simulink model "AuM_HA_05_A2"  (R2020a)
settings: Solver=VariableStepAuto  StartTime=0.0  StopTime=0.2  FixedStep=1e-8  MaxStep=1e-4  MinStep=1e-9  RelTol=1e-10  EnableMultiTasking=on
values from neighbouring files (symbols this model uses):
  f_PWM = 16000    [AuM_HA05_A1_init.m]    (also in AuM_HA05_A2_init.m)
  J = 450e-6    (= 0.00045)    [AuM_HA05_A1_init.m]    (also in AuM_HA05_A2_init.m)
  K_pi = (T_oi.^2+T_S.^2)/(2/R_S*T_oi*T_S)    [AuM_HA05_A1_init.m]    (also in AuM_HA05_A2_init.m)
  L_S = 4e-3    (= 0.004)    [AuM_HA05_A1_init.m]    (also in AuM_HA05_A2_init.m)
  p = 5    [AuM_HA05_A1_init.m]    (also in AuM_HA05_A2_init.m)
  Psi_P = 4.5e-3    (= 0.0045)    [AuM_HA05_A1_init.m]    (also in AuM_HA05_A2_init.m)
  R_S = 0.58    [AuM_HA05_A1_init.m]    (also in AuM_HA05_A2_init.m)
  T_mi = 50e-6    (= 5e-05)    [AuM_HA05_A1_init.m]    (also in AuM_HA05_A2_init.m)
  T_mw = 908e-6    (= 0.000908)    [AuM_HA05_A1_init.m]    (also in AuM_HA05_A2_init.m)
  T_ni = 4*T_oi*T_S*(T_oi.^2+T_S.^2)/(T_oi+T_S).^3    [AuM_HA05_A1_init.m]    (also in AuM_HA05_A2_init.m)
  T_S = L_S/R_S    (= 0.00689655172414)    [AuM_HA05_A1_init.m]    (also in AuM_HA05_A2_init.m)
  T_SR = 50e-6    (= 5e-05)    [AuM_HA05_A1_init.m]    (also in AuM_HA05_A2_init.m)
  U_d = 24    [AuM_HA05_A1_init.m]    (also in AuM_HA05_A2_init.m)
undefined symbols (not defined in the file or in its folder): magnitude
libraries: simulink x1
settings Model: Creator=junglas  LastModifiedBy=Ravi Plenzdorf
settings SolverCC: MaxConsecutiveZCs=10000  ZeroCrossAlgorithm=Adaptive
settings DataIOCC: ReturnWorkspaceOutputs=off
settings OptimizationCC: LifeSpan=inf
settings DebuggingCC: SFUnexpectedBacktrackingDiag=warning  SFNoUnconditionalDefaultTransitionDiag=warning  SFExecutionAtInitializationDiag=none  ArithmeticOperatorsInVariantConditions=warning
settings SFSimCC: SimUseLocalCustomCode=off  CustomCodeUndefinedFunction=UseInterfaceOnly
settings RTWCC: RTWUseLocalCustomCode=off
settings CodeAppCC: StateflowObjectComments=on
settings GRTTargetCC: TargetLangStandard=C89/C90 (ANSI)
settings ConfigComp: CovMetricSettings=dw  CovHtmlReporting=on  CovSaveCumulativeToWorkspaceVar=on  CovSaveSingleToWorkspaceVar=on  CovExternalEMLEnable=off

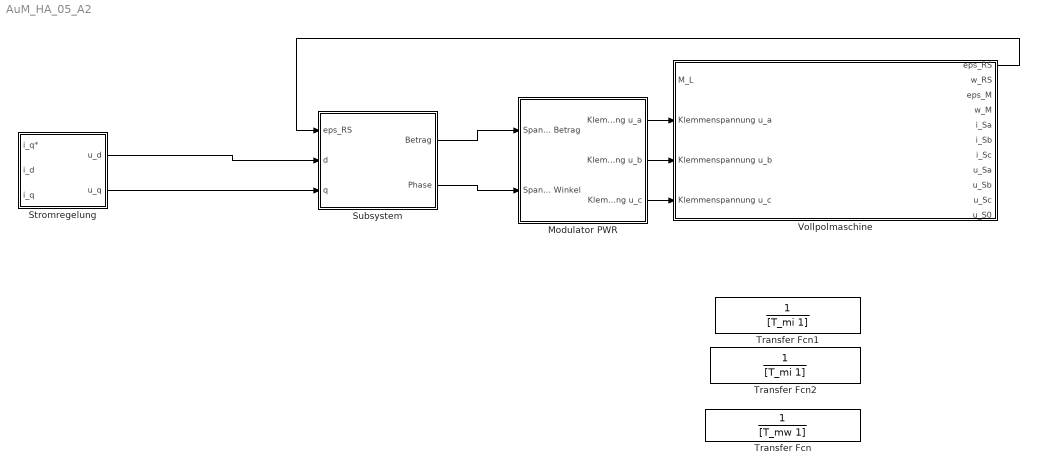
== system AuM_HA_05_A2 ==
  Modulator PWR : Subsystem  SystemSampleTime=1/1e6
  Stromregelung : Subsystem
  Subsystem : Subsystem
  Transfer Fcn : TransferFcn  Denominator=[T_mw 1]
  Transfer Fcn1 : TransferFcn  Denominator=[T_mi 1]
  Transfer Fcn2 : TransferFcn  Denominator=[T_mi 1]
  Vollpolmaschine : Subsystem
      mask Display: image('Motor_Symbol.png'); % Use "Edit Image" on toolstrip to change.
  wires:
  Modulator PWR/1(Klemmenspannung u_a) -> Vollpolmaschine/2(Klemmenspannung u_a)
  Modulator PWR/2(Klemmenspannung u_b) -> Vollpolmaschine/3(Klemmenspannung u_b)
  Modulator PWR/3(Klemmenspannung u_c) -> Vollpolmaschine/4(Klemmenspannung u_c)
  Vollpolmaschine/1(eps_RS) -> Subsystem/1(eps_RS)
  Stromregelung/1(u_d) -> Subsystem/2(d)
  Stromregelung/2(u_q) -> Subsystem/3(q)
  Subsystem/2(Phase) -> Modulator PWR/2(Spannung Winkel)
  Subsystem/1(Betrag) -> Modulator PWR/1(Spannung Betrag)

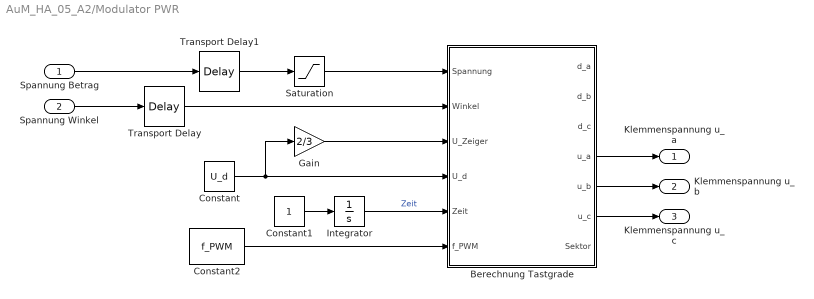
== system AuM_HA_05_A2/Modulator PWR ==
  Spannung Betrag : Inport
  Spannung Winkel : Inport  Port=2
  Berechnung Tastgrade : MATLAB Function  SystemSampleTime=1e-6
  Constant : Constant  Value=U_d
  Constant1 : Constant
  Constant2 : Constant  Value=f_PWM
  Gain : Gain  Gain=2/3
  Integrator : Integrator
  Saturation : Saturate  UpperLimit=U_d*sqrt(3)/2  LowerLimit=0
  Transport Delay : TransportDelay  DelayTime=T_SR
  Transport Delay1 : TransportDelay  DelayTime=T_SR
  Klemmenspannung u_a : Outport  VectorParamsAs1DForOutWhenUnconnected=off
  Klemmenspannung u_b : Outport  Port=2  VectorParamsAs1DForOutWhenUnconnected=off
  Klemmenspannung u_c : Outport  Port=3  VectorParamsAs1DForOutWhenUnconnected=off
  wires:
  Spannung Betrag/1 -> Transport Delay1/1
  Integrator/1 -> Berechnung Tastgrade/5(Zeit)  "Zeit"
  Constant/1 -> Berechnung Tastgrade/4(U_d), Gain/1
  Gain/1 -> Berechnung Tastgrade/3(U_Zeiger)
  Berechnung Tastgrade/6(u_c) -> Klemmenspannung u_c/1
  Berechnung Tastgrade/5(u_b) -> Klemmenspannung u_b/1
  Berechnung Tastgrade/4(u_a) -> Klemmenspannung u_a/1
  Saturation/1 -> Berechnung Tastgrade/1(Spannung)
  Constant1/1 -> Integrator/1
  Constant2/1 -> Berechnung Tastgrade/6(f_PWM)
  Spannung Winkel/1 -> Transport Delay/1
  Transport Delay/1 -> Berechnung Tastgrade/2(Winkel)
  Transport Delay1/1 -> Saturation/1

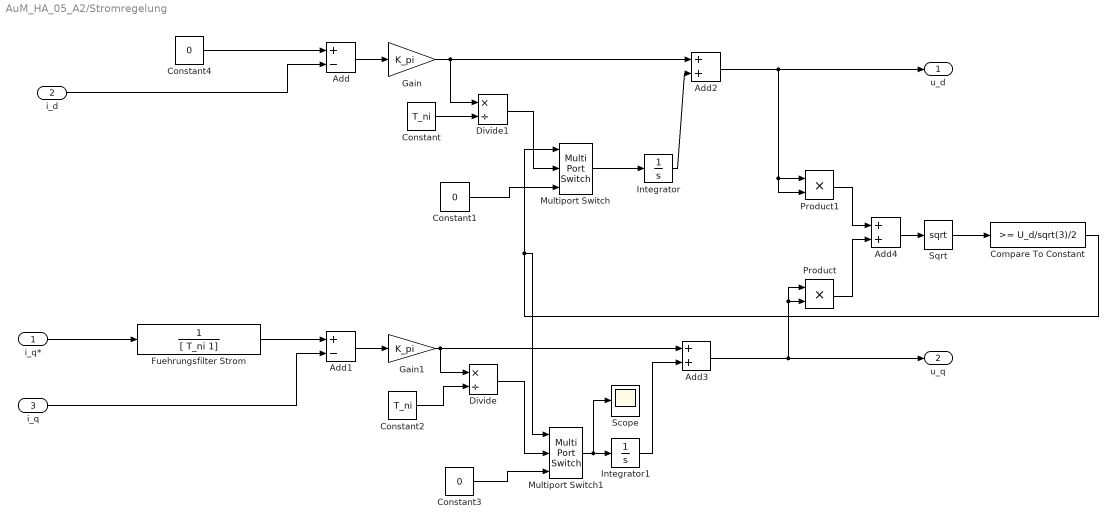
== system AuM_HA_05_A2/Stromregelung ==
  i_q* : Inport
  i_d : Inport  Port=2
  i_q : Inport  Port=3
  Add : Sum  Inputs=+-
  Add1 : Sum  Inputs=+-
  Add2 : Sum
  Add3 : Sum
  Add4 : Sum
  Compare To Constant : simulink/Logic and Bit Operations/Compare To Constant  relop=>=  const=U_d/sqrt(3)/2  OutDataTypeStr=boolean
  Constant : Constant  Value=T_ni
  Constant1 : Constant  Value=0
  Constant2 : Constant  Value=T_ni
  Constant3 : Constant  Value=0
  Constant4 : Constant  Value=0
  Divide : Product  Inputs=*/
  Divide1 : Product  Inputs=*/
  Fuehrungsfilter Strom : TransferFcn  Denominator=[ T_ni 1]
  Gain : Gain  Gain=K_pi
  Gain1 : Gain  Gain=K_pi
  Integrator : Integrator
  Integrator1 : Integrator
  Multiport Switch : MultiPortSwitch  DataPortOrder=Specify indices  DataPortIndices={0,1}
  Multiport Switch1 : MultiPortSwitch  DataPortOrder=Specify indices  DataPortIndices={0,1}
  Product : Product
  Product1 : Product
  Scope : Scope
  Sqrt : Sqrt  SaturateOnIntegerOverflow=on
  u_d : Outport  VectorParamsAs1DForOutWhenUnconnected=off
  u_q : Outport  Port=2  VectorParamsAs1DForOutWhenUnconnected=off
  wires:
  i_q/1 -> Add1/2
  i_d/1 -> Add/2
  Add1/1 -> Gain1/1
  Add/1 -> Gain/1
  i_q*/1 -> Fuehrungsfilter Strom/1
  Gain/1 -> Add2/1, Divide1/1
  Integrator/1 -> Add2/2
  Integrator1/1 -> Add3/2
  Gain1/1 -> Divide/1, Add3/1
  Constant/1 -> Divide1/2
  Multiport Switch/1 -> Integrator/1
  Constant2/1 -> Divide/2
  Multiport Switch1/1 -> Scope/1, Integrator1/1
  Add2/1 -> Product1/2, Product1/1, u_d/1
  Add3/1 -> Product/1, Product/2, u_q/1
  Constant4/1 -> Add/1
  Constant3/1 -> Multiport Switch1/3
  Divide/1 -> Multiport Switch1/2
  Divide1/1 -> Multiport Switch/2
  Constant1/1 -> Multiport Switch/3
  Compare To Constant/1 -> Multiport Switch1/1, Multiport Switch/1
  Fuehrungsfilter Strom/1 -> Add1/1
  Product/1 -> Add4/2
  Product1/1 -> Add4/1
  Add4/1 -> Sqrt/1
  Sqrt/1 -> Compare To Constant/1

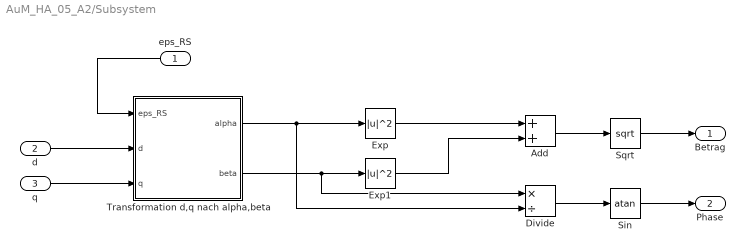
== system AuM_HA_05_A2/Subsystem ==
  eps_RS : Inport
  d : Inport  Port=2
  q : Inport  Port=3
  Add : Sum
  Divide : Product  Inputs=*/
  Exp : Math  Operator=magnitude^2  SaturateOnIntegerOverflow=on
  Exp1 : Math  Operator=magnitude^2  SaturateOnIntegerOverflow=on
  Sin : Trigonometry  Operator=atan
  Sqrt : Sqrt  SaturateOnIntegerOverflow=on
  Transformation d,q nach alpha,beta : MATLAB Function  TreatAsAtomicUnit=on
  Betrag : Outport
  Phase : Outport  Port=2
  wires:
  Exp1/1 -> Add/2
  Transformation d,q nach alpha,beta/2(beta) -> Exp1/1, Divide/1
  Transformation d,q nach alpha,beta/1(alpha) -> Divide/2, Exp/1
  Exp/1 -> Add/1
  Add/1 -> Sqrt/1
  eps_RS/1 -> Transformation d,q nach alpha,beta/1(eps_RS)
  q/1 -> Transformation d,q nach alpha,beta/3(q)
  d/1 -> Transformation d,q nach alpha,beta/2(d)
  Sqrt/1 -> Betrag/1
  Divide/1 -> Sin/1
  Sin/1 -> Phase/1

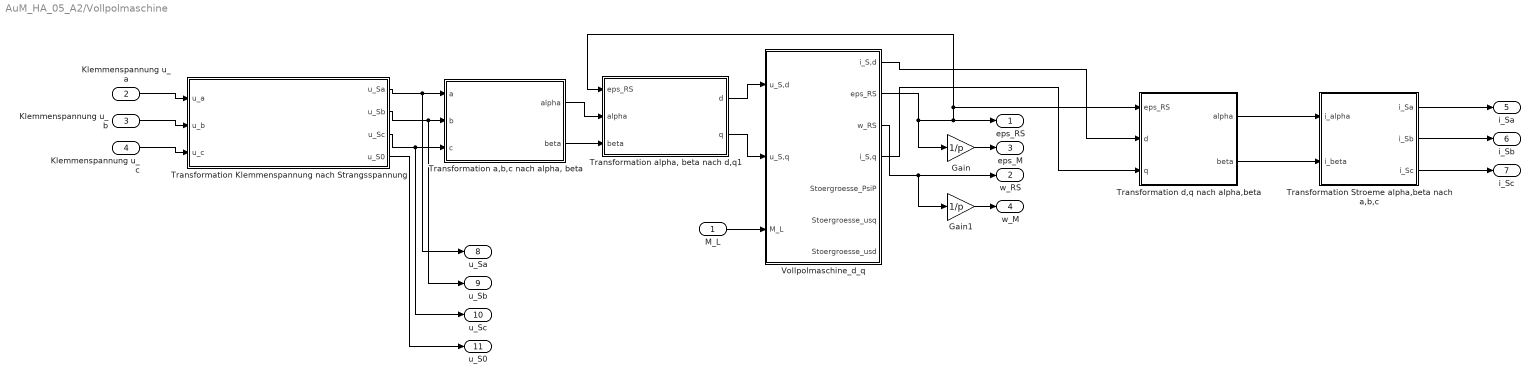
== system AuM_HA_05_A2/Vollpolmaschine ==
  M_L : Inport
  Klemmenspannung u_a : Inport  Port=2
  Klemmenspannung u_b : Inport  Port=3
  Klemmenspannung u_c : Inport  Port=4
  Gain : Gain  Gain=1/p
  Gain1 : Gain  Gain=1/p
  Transformation Klemmenspannung nach Strangsspannung : MATLAB Function  TreatAsAtomicUnit=on
  Transformation Stroeme alpha,beta nach a,b,c : MATLAB Function  TreatAsAtomicUnit=on
  "Transformation a,b,c nach alpha, beta" : MATLAB Function  TreatAsAtomicUnit=on
  "Transformation alpha, beta nach d,q1" : MATLAB Function  TreatAsAtomicUnit=on
  Transformation d,q nach alpha,beta : MATLAB Function  TreatAsAtomicUnit=on
  Vollpolmaschine_d_q : Subsystem
  eps_RS : Outport  VectorParamsAs1DForOutWhenUnconnected=off
  w_RS : Outport  Port=2  VectorParamsAs1DForOutWhenUnconnected=off
  eps_M : Outport  Port=3  VectorParamsAs1DForOutWhenUnconnected=off
  w_M : Outport  Port=4  VectorParamsAs1DForOutWhenUnconnected=off
  i_Sa : Outport  Port=5  VectorParamsAs1DForOutWhenUnconnected=off
  i_Sb : Outport  Port=6  VectorParamsAs1DForOutWhenUnconnected=off
  i_Sc : Outport  Port=7  VectorParamsAs1DForOutWhenUnconnected=off
  u_Sa : Outport  Port=8  VectorParamsAs1DForOutWhenUnconnected=off
  u_Sb : Outport  Port=9  VectorParamsAs1DForOutWhenUnconnected=off
  u_Sc : Outport  Port=10  VectorParamsAs1DForOutWhenUnconnected=off
  u_S0 : Outport  Port=11  VectorParamsAs1DForOutWhenUnconnected=off
  wires:
  Vollpolmaschine_d_q/4(i_S,q) -> Transformation d,q nach alpha,beta/3(q)
  Vollpolmaschine_d_q/1(i_S,d) -> Transformation d,q nach alpha,beta/2(d)
  Transformation Klemmenspannung nach Strangsspannung/2(u_Sb) -> u_Sb/1, "Transformation a,b,c nach alpha, beta"/2(b)
  Vollpolmaschine_d_q/3(w_RS) -> Gain1/1, w_RS/1
  Transformation Klemmenspannung nach Strangsspannung/1(u_Sa) -> u_Sa/1, "Transformation a,b,c nach alpha, beta"/1(a)
  Vollpolmaschine_d_q/2(eps_RS) -> eps_RS/1, Transformation d,q nach alpha,beta/1(eps_RS), "Transformation alpha, beta nach d,q1"/1(eps_RS), Gain/1
  Transformation Klemmenspannung nach Strangsspannung/3(u_Sc) -> "Transformation a,b,c nach alpha, beta"/3(c), u_Sc/1
  M_L/1 -> Vollpolmaschine_d_q/3(M_L)
  "Transformation a,b,c nach alpha, beta"/1(alpha) -> "Transformation alpha, beta nach d,q1"/2(alpha)
  "Transformation a,b,c nach alpha, beta"/2(beta) -> "Transformation alpha, beta nach d,q1"/3(beta)
  "Transformation alpha, beta nach d,q1"/2(q) -> Vollpolmaschine_d_q/2(u_S,q)
  Klemmenspannung u_a/1 -> Transformation Klemmenspannung nach Strangsspannung/1(u_a)
  Klemmenspannung u_b/1 -> Transformation Klemmenspannung nach Strangsspannung/2(u_b)
  Klemmenspannung u_c/1 -> Transformation Klemmenspannung nach Strangsspannung/3(u_c)
  Gain/1 -> eps_M/1
  Gain1/1 -> w_M/1
  "Transformation alpha, beta nach d,q1"/1(d) -> Vollpolmaschine_d_q/1(u_S,d)
  Transformation d,q nach alpha,beta/1(alpha) -> Transformation Stroeme alpha,beta nach a,b,c/1(i_alpha)
  Transformation d,q nach alpha,beta/2(beta) -> Transformation Stroeme alpha,beta nach a,b,c/2(i_beta)
  Transformation Stroeme alpha,beta nach a,b,c/1(i_Sa) -> i_Sa/1
  Transformation Stroeme alpha,beta nach a,b,c/2(i_Sb) -> i_Sb/1
  Transformation Stroeme alpha,beta nach a,b,c/3(i_Sc) -> i_Sc/1
  Transformation Klemmenspannung nach Strangsspannung/4(u_S0) -> u_S0/1

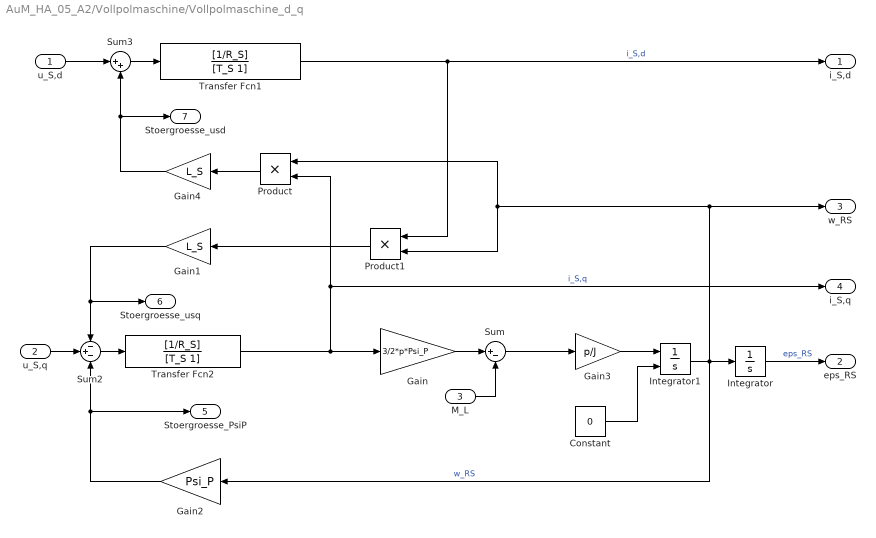
== system AuM_HA_05_A2/Vollpolmaschine/Vollpolmaschine_d_q ==
  u_S,d : Inport
  u_S,q : Inport  Port=2
  M_L : Inport  Port=3
  Constant : Constant  Value=0
  Gain : Gain  Gain=3/2*p*Psi_P
  Gain1 : Gain  Gain=L_S
  Gain2 : Gain  Gain=Psi_P
  Gain3 : Gain  Gain=p/J
  Gain4 : Gain  Gain=L_S
  Integrator : Integrator
  Integrator1 : Integrator  InitialConditionSource=external
  Product : Product
  Product1 : Product
  Sum : Sum  Inputs=|+-
  Sum2 : Sum  Inputs=-+-
  Sum3 : Sum  Inputs=|++
  Transfer Fcn1 : TransferFcn  Numerator=[1/R_S]  Denominator=[T_S 1]
  Transfer Fcn2 : TransferFcn  Numerator=[1/R_S]  Denominator=[T_S 1]
  i_S,d : Outport  VectorParamsAs1DForOutWhenUnconnected=off
  eps_RS : Outport  Port=2  VectorParamsAs1DForOutWhenUnconnected=off
  w_RS : Outport  Port=3  VectorParamsAs1DForOutWhenUnconnected=off
  i_S,q : Outport  Port=4  VectorParamsAs1DForOutWhenUnconnected=off
  Stoergroesse_PsiP : Outport  Port=5  VectorParamsAs1DForOutWhenUnconnected=off
  Stoergroesse_usq : Outport  Port=6  VectorParamsAs1DForOutWhenUnconnected=off
  Stoergroesse_usd : Outport  Port=7  VectorParamsAs1DForOutWhenUnconnected=off
  wires:
  Sum2/1 -> Transfer Fcn2/1
  Integrator1/1 -> Integrator/1, w_RS/1, Product/1, Product1/2, Gain2/1  "w_RS"
  Integrator/1 -> eps_RS/1  "eps_RS"
  Sum/1 -> Gain3/1
  M_L/1 -> Sum/2
  Gain/1 -> Sum/1
  Gain3/1 -> Integrator1/1
  Gain2/1 -> Stoergroesse_PsiP/1, Sum2/3
  Sum3/1 -> Transfer Fcn1/1
  Product/1 -> Gain4/1
  Transfer Fcn1/1 -> i_S,d/1, Product1/1  "i_S,d"
  Product1/1 -> Gain1/1
  u_S,q/1 -> Sum2/2
  Gain1/1 -> Stoergroesse_usq/1, Sum2/1
  u_S,d/1 -> Sum3/1
  Gain4/1 -> Stoergroesse_usd/1, Sum3/2
  Transfer Fcn2/1 -> Gain/1, i_S,q/1, Product/2  "i_S,q"
  Constant/1 -> Integrator1/2

== matlab function AuM_HA_05_A2/Subsystem/Transformation d,q nach alpha,beta ==
  data: eps_RS input; alpha output; d input; q input; beta output
function [alpha,beta] = fcn(eps_RS,d,q)
%#codegen
In=[d;q];
Out=[cos(eps_RS) -sin(eps_RS);sin(eps_RS) cos(eps_RS)]*In;
alpha=Out(1);
beta=Out(2);

== matlab function AuM_HA_05_A2/Vollpolmaschine/Transformation d,q nach alpha,beta ==
  data: eps_RS input; alpha output; d input; q input; beta output
function [alpha,beta] = fcn(eps_RS,d,q)
%#codegen
In=[d;q];
Out=[cos(eps_RS) -sin(eps_RS);sin(eps_RS) cos(eps_RS)]*In;
alpha=Out(1);
beta=Out(2);

== matlab function AuM_HA_05_A2/Vollpolmaschine/Transformation Stroeme alpha,beta nach a,b,c ==
  data: i_alpha input; i_Sa output; i_beta input; i_Sb output; i_Sc output
function [i_Sa,i_Sb,i_Sc] = fcn(i_alpha,i_beta)
%#codegen
In=[i_alpha;i_beta];
Mat=[1 0; -0.5 sqrt(3)/2];
Out=Mat*In;
i_Sa=Out(1);
i_Sb=Out(2);
i_Sc=-i_Sa-i_Sb;

== matlab function AuM_HA_05_A2/Modulator PWR/Berechnung Tastgrade ==
  data: Spannung input; d_a output; Winkel input; d_b output; d_c output; U_Zeiger input; U_d input; Zeit input; u_a output; u_b output; u_c output; Sektor output; f_PWM input
function [d_a,d_b,d_c,u_a,u_b,u_c,Sektor]= fcn(Spannung, Winkel,U_Zeiger,U_d, Zeit, f_PWM)

%Winkel auf 0 bis 2pi bringen

while Winkel>=2*pi
    Winkel=Winkel-2*pi;
end
while Winkel<0
    Winkel=Winkel+2*pi;
end

%Winkel dekrementieren, bis er sich zwischen 0 und 60 Grad befindet
Sektor=1;
while Winkel>pi/3
    Sektor=Sektor+1;
    Winkel=Winkel-pi/3;
end
%Zeiger berechnen
Zeigerlaenge_2_normiert=sin(Winkel)/sin(pi/3)*Spannung/U_Zeiger;
Zeigerlaenge_1_normiert=cos(Winkel)*Spannung/U_Zeiger-cos(pi/3)*Zeigerlaenge_2_normiert;
Nullzeiger=1-Zeigerlaenge_2_normiert-Zeigerlaenge_1_normiert;

switch Sektor
    case 1
        d_a=Nullzeiger/2+Zeigerlaenge_2_normiert+Zeigerlaenge_1_normiert;
        d_b=Nullzeiger/2+Zeigerlaenge_2_normiert;
        d_c=Nullzeiger/2;
    case 2
        d_a=Nullzeiger/2+Zeigerlaenge_1_normiert;
        d_b=Nullzeiger/2+Zeigerlaenge_1_normiert+Zeigerlaenge_2_normiert;
        d_c=Nullzeiger/2;
    case 3
        d_b=Nullzeiger/2+Zeigerlaenge_2_normiert+Zeigerlaenge_1_normiert;
        d_c=Nullzeiger/2+Zeigerlaenge_2_normiert;
        d_a=Nullzeiger/2;
    case 4
        d_b=Nullzeiger/2+Zeigerlaenge_1_normiert;
        d_c=Nullzeiger/2+Zeigerlaenge_1_normiert+Zeigerlaenge_2_normiert;
        d_a=Nullzeiger/2;
    case 5
        d_c=Nullzeiger/2+Zeigerlaenge_2_normiert+Zeigerlaenge_1_normiert;
        d_a=Nullzeiger/2+Zeigerlaenge_2_normiert;
        d_b=Nullzeiger/2;
    case 6
        d_c=Nullzeiger/2+Zeigerlaenge_1_normiert;
        d_a=Nullzeiger/2+Zeigerlaenge_1_normiert+Zeigerlaenge_2_normiert;
        d_b=Nullzeiger/2;
    otherwise
        d_a=0.5;
        d_b=0.5;
        d_c=0.5;
end

Rest_Zeit=(floor(Zeit*f_PWM))/f_PWM;
Zeit_in_PWM_Intervall=Zeit-Rest_Zeit;
Vergleichswert=abs(Zeit_in_PWM_Intervall*f_PWM*2-1);

if d_a>Vergleichswert
    u_a=U_d;
else
    u_a=0;
end



if d_b>Vergleichswert
    u_b=U_d;
else
    u_b=0;
end

if d_c>Vergleichswert
    u_c=U_d;
else
    u_c=0;
end

== matlab function AuM_HA_05_A2/Vollpolmaschine/Transformation Klemmenspannung nach Strangsspannung ==
  data: u_a input; u_Sa output; u_b input; u_c input; u_Sb output; u_Sc output; u_S0 output
function [u_Sa,u_Sb,u_Sc,u_S0] = fcn(u_a,u_b,u_c)
%Konvertiert Klemmenspannungen in Strangspannungen
u_S0=u_a/3+u_b/3+u_c/3;
u_Sa=u_a-u_S0;
u_Sb=u_b-u_S0;
u_Sc=u_c-u_S0;
end

== matlab function AuM_HA_05_A2/Vollpolmaschine/Transformation a,b,c nach alpha, beta ==
  data: a input; alpha output; b input; c input; beta output
function [alpha,beta] = fcn(a,b,c)
In=[a;b;c];
Out=2/3*[1 -0.5 -0.5; 0 sqrt(3)/2 -sqrt(3)/2]*In;
alpha=Out(1);
beta=Out(2);

== matlab function AuM_HA_05_A2/Vollpolmaschine/Transformation alpha, beta nach d,q1 ==
  data: eps_RS input; d output; alpha input; beta input; q output
function [d,q] = fcn(eps_RS,alpha,beta)
%#codegen
In=[alpha;beta];
Out=[cos(eps_RS) sin(eps_RS);-sin(eps_RS) cos(eps_RS)]*In;
d=Out(1);
q=Out(2);
